simulink model "SysTheoryNo4Model"  (R2023a)
settings: Solver=VariableStepAuto  StartTime=0.0  StopTime=sysTime  RelTol=1e-3
values from neighbouring files (symbols this model uses):
  M0 = 3    [SysTheoryNo4.m]
  M1 = 10    [SysTheoryNo4.m]
  M2 = pi / 4    (= 0.785398163397)    [SysTheoryNo4.m]
  sysA = double(subs(symA, paramArray, paramValues{paramChoise}))    [SysTheoryNo3.m]    (also in SysTheoryNo4.m)
  sysAnoise = double(subs(symA, paramArray, paramValuesNoise))    [SysTheoryNo3.m]    (also in SysTheoryNo4.m)
  sysAsinfinal = [ ... (first row only)    [SysTheoryNo4.m]
  sysB = double(subs(symB, paramArray, paramValues{paramChoise}))    [SysTheoryNo3.m]    (also in SysTheoryNo4.m)
  sysBnoise = double(subs(symB, paramArray, paramValuesNoise))    [SysTheoryNo3.m]    (also in SysTheoryNo4.m)
  sysBsinfinal = [ ... (first row only)    [SysTheoryNo4.m]
  sysC = [ ... (first row only)    [SysTheoryNo3.m]    (also in SysTheoryNo4.m)
  sysCsinfinal = [zeros(size(sysCsin)), 0, 1]    [SysTheoryNo4.m]
  sysD = 0    [SysTheoryNo3.m]    (also in SysTheoryNo4.m)
  sysDsinfinal = zeros(size(sysDsin))    [SysTheoryNo4.m]
  sysF = - Pi * polyvalm(double(sym2poly(pAFeedback)), transpose(sysA))    [SysTheoryNo3.m]
  sysInit = [q1Init; q2Init; dq1Init; dq2Init]    [SysTheoryNo3.m]    (also in SysTheoryNo4.m)
  sysV = transpose(sysV)    [SysTheoryNo4.m]
settings Model: Creator=utente  LastModifiedBy=utente

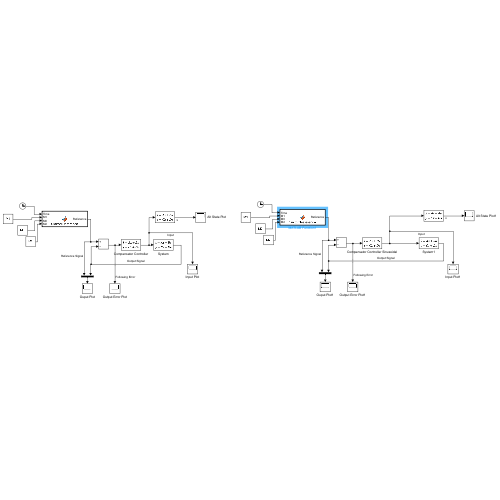
[thumbnail: Simulink's stored preview of the top-level diagram]
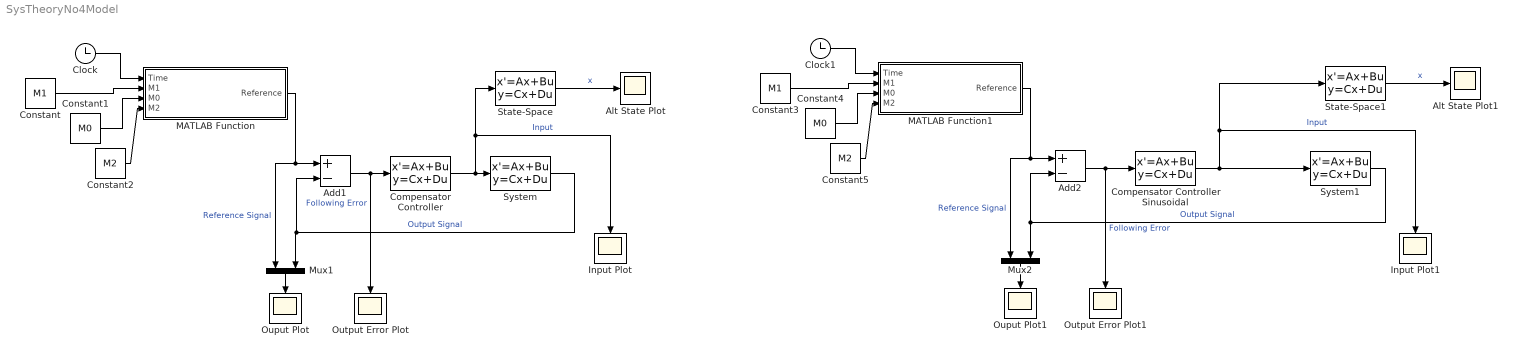
== system SysTheoryNo4Model ==
  Add1 : Sum  Inputs=+-
  Add2 : Sum  Inputs=+-
  Alt State Plot : Scope
  Alt State Plot1 : Scope
  Clock : Clock
  Clock1 : Clock
  Compensator Controller : StateSpace  A=sysA - sysV * sysC + sysB * sysF - sysV * sysD * sysF  B=- sysV  C=sysF  D=0  InitialCondition=zeros(4, 1)
  Compensator Controller Sinusoidal : StateSpace  A=sysAsinfinal  B=sysBsinfinal  C=sysCsinfinal  D=sysDsinfinal  InitialCondition=zeros(8, 1)
  Constant : Constant  Value=M1
  Constant1 : Constant  Value=M0
  Constant2 : Constant  Value=M2
  Constant3 : Constant  Value=M1
  Constant4 : Constant  Value=M0
  Constant5 : Constant  Value=M2
  Input Plot : Scope
  Input Plot1 : Scope
  MATLAB Function : MATLAB Function  TreatAsAtomicUnit=on
  MATLAB Function1 : MATLAB Function  TreatAsAtomicUnit=on
  Mux1 : Mux  Inputs=2
  Mux2 : Mux  Inputs=2
  Ouput Plot : Scope
  Ouput Plot1 : Scope
  Output Error Plot : Scope
  Output Error Plot1 : Scope
  State-Space : StateSpace  A=sysAnoise  B=sysBnoise  C=eye(4)  D=sysD * zeros(4, 1)  InitialCondition=sysInit
  State-Space1 : StateSpace  A=sysAnoise  B=sysBnoise  C=eye(4)  D=sysD * zeros(4, 1)  InitialCondition=sysInit
  System : StateSpace  A=sysAnoise  B=sysBnoise  C=sysC  D=sysD  InitialCondition=sysInit
  System1 : StateSpace  A=sysAnoise  B=sysBnoise  C=sysC  D=sysD  InitialCondition=sysInit
  wires:
  System/1 -> Mux1/2, Add1/2  "Output Signal"
  MATLAB Function/1(Reference) -> Mux1/1, Add1/1  "Reference Signal"
  Compensator Controller/1 -> Input Plot/1, State-Space/1, System/1  "Input"
  Mux1/1 -> Ouput Plot/1
  Add1/1 -> Compensator Controller/1, Output Error Plot/1  "Following Error"
  State-Space/1 -> Alt State Plot/1  "x"
  Clock/1 -> MATLAB Function/1(Time)
  Constant/1 -> MATLAB Function/2(M1)
  Constant1/1 -> MATLAB Function/3(M0)
  Constant2/1 -> MATLAB Function/4(M2)
  Clock1/1 -> MATLAB Function1/1(Time)
  Constant4/1 -> MATLAB Function1/3(M0)
  Constant3/1 -> MATLAB Function1/2(M1)
  MATLAB Function1/1(Reference) -> Mux2/1, Add2/1  "Reference Signal"
  System1/1 -> Add2/2, Mux2/2  "Output Signal"
  Add2/1 -> Compensator Controller Sinusoidal/1, Output Error Plot1/1  "Following Error"
  Constant5/1 -> MATLAB Function1/4(M2)
  Compensator Controller Sinusoidal/1 -> System1/1, State-Space1/1, Input Plot1/1  "Input"
  Mux2/1 -> Ouput Plot1/1
  State-Space1/1 -> Alt State Plot1/1  "x"

== matlab function SysTheoryNo4Model/MATLAB Function1 ==
  data: Time input; Reference output; M1 input; M0 input; M2 input
function Reference = CustomReference(Time, M1, M0, M2)
if(Time < 100)
    Reference = M1 * Time + M0;
elseif(Time < 200)
    Reference = M0;
elseif(Time < 300)
    Reference = M1;
else
    Reference = M1 * sin(M0 * Time + M2);
end

== matlab function SysTheoryNo4Model/MATLAB Function ==
  data: Time input; Reference output; M1 input; M0 input; M2 input
function Reference = CustomReference(Time, M1, M0, M2)
if(Time < 100)
    Reference = M1 * Time + M0;
elseif(Time < 200)
    Reference = M0;
elseif(Time < 300)
    Reference = M1;
else
    Reference = M1 * sin(M0 * Time + M2);
end
